simulink model "Scissor_Lift_2_Spring_Actuation"  (Simulink 7.9)
settings: Solver=ode15s  StartTime=0.0  StopTime=10.0  MaxStep=1e-2  RelTol=1e-3  AbsTol=1e-4
PostLoadFcn:
  | warning off mech2:compiler:topologyAnalysis:DanglingBlock
undefined symbols (not defined in the file): Local, Scissor_Lift_Param, X, Y, Z
libraries: sm_lib x46, Scissor_Parts_Lib x22, nesl_utility x3
(part 1 of 2)
Description:
  | Copyright 2012 The MathWorks, Inc.
settings Model: Creator=smiller  LastModifiedBy=smiller
settings ConfigurationSet: Description=SimMechanics 2G
settings ExplorerConfigSet: InternalSimMechanicsExplorerSettings="<ExplorerConfiguration><canonicalview>default</canonicalview><TilePanel><TileInfo><Tiles Columns=\"1\" Count=\"1\" Rows=\"1\"><Column Left=\"2\" Weight=\"1\"/><Column Left=\"398\"/><Row Top=\"2\" Weight=\"1\"/><Row Top=\"485\"/><Tile Height=\"1\" Width=\"1\" X=\"0\" Y=\"0\"/></Tiles></TileInfo><SceneInfo><SceneViewer><BGColor><R>0.60000002384185791</R><G>0.60000002384185791</G><B>0.60000002384185791</B></BGColor><Camera><Position><X>5.9281055778528522</X><Y>-5.497525414498786</Y><Z>4.0727654141199023</Z></Position><Center><X>1.3999999761581421</X><Y>0</Y><Z>1.5331412553787231</Z></Center><Up><X>-0.23055989473784222</X><Y>0.24511291789662082</Y><Z>0.94168030266045166</Z></Up><Left>-1.6471169292926788</Left><Right>1.6471169292926788</Right><Bottom>-2.5798462629318237</Bottom><Top>2.5798462629318237</Top></Camera></SceneViewer></SceneInfo></TilePanel></ExplorerConfiguration>"

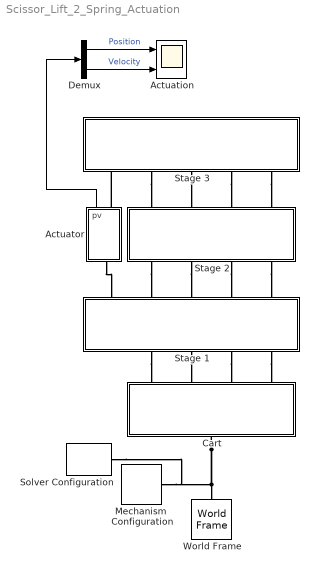
== system Scissor_Lift_2_Spring_Actuation ==
  Actuation : Scope  NumInputPorts=2
      settings: TimeRange=10  YMin=1.744052650646057~-0.2  YMax=2.541057843255645~0.3  SaveName=ScopeData3
  Actuator : Subsystem
  Cart : Subsystem
  Demux : Demux  Outputs=2
  Mechanism  Configuration : sm_lib/Utilities/Mechanism  Configuration  GravityVector=[0 0 -9.81]  GravityUnits=m/s^2  AllowGravitySignal=off  LinearizationDelta=0.001  BlockFunction=simmechanics.library.utilities.mechanism_configuration
  Solver Configuration : nesl_utility/Solver Configuration  PhysicalDomain=network_engine_domain  LeftPortType=input  RightPortType=generic  SubClassName=solver  UseCustomDae=off  DoDC=off  ResidualTolerance=1e-9  UseLocalSolver=off  LocalSolverChoice=NE_BACKWARD_EULER_ADVANCER  LocalSolverSampleTime=.001  DoFixedCost=off  MaxNonlinIter=3  MaxModeIter=2  LinearAlgebra=Sparse  Accelerate=off  Profile=off  UseLocalSampling=off  DelaysMemoryBudget=1024
  Stage 1 : Subsystem
  Stage 2 : Subsystem
  Stage 3 : Subsystem
  World Frame : sm_lib/Frames and  Transforms/World Frame  BlockFunction=simmechanics.library.frames_transforms.world_frame
  wires:
  Demux/1 -> Actuation/1  "Position"
  Demux/2 -> Actuation/2  "Velocity"
  Actuator/1(pv) -> Demux/1
  connections:
  Cart/LConn1 -- World Frame/RConn1 -- Solver Configuration/RConn1 -- Mechanism  Configuration/RConn1
  Stage 2/RConn1 -- Stage 1/LConn2
  Stage 2/RConn4 -- Stage 1/LConn5
  Stage 3/RConn2 -- Stage 2/LConn1
  Stage 2/RConn3 -- Stage 1/LConn4
  Stage 3/RConn4 -- Stage 2/LConn3
  Stage 3/RConn5 -- Stage 2/LConn4
  Stage 3/RConn3 -- Stage 2/LConn2
  Stage 1/RConn4 -- Cart/RConn3
  Stage 1/RConn3 -- Cart/RConn2
  Actuator/RConn1 -- Stage 3/RConn1
  Actuator/LConn1 -- Stage 1/LConn1
  Stage 1/RConn2 -- Cart/RConn1
  Stage 2/RConn2 -- Stage 1/LConn3
  Stage 1/RConn5 -- Cart/RConn4

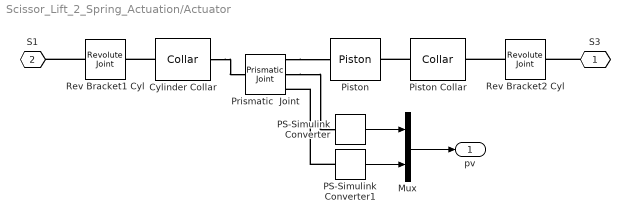
== system Scissor_Lift_2_Spring_Actuation/Actuator ==
  Cylinder Collar : Scissor_Parts_Lib/Collar  collar_length=Scissor_Lift_Param.Actuator.Collar.Length  collar_radius=Scissor_Lift_Param.Actuator.Collar.Radius  cylinder_length=Scissor_Lift_Param.Actuator.Cylinder.Length  cylinder_radius=Scissor_Lift_Param.Actuator.Cylinder.Radius  cylinder_ori=Local +Z  material_density=Scissor_Lift_Param.Actuator.Collar.Density  material_color=Scissor_Lift_Param.Actuator.Collar.Color  material_opacity=Scissor_Lift_Param.Actuator.Collar.Opacity
  Mux : Mux  Inputs=2
  PS-Simulink Converter : nesl_utility/PS-Simulink Converter  PhysicalDomain=network_engine_domain  LeftPortType=input  RightPortType=output  SubClassName=ps_output  Unit=1  AffineConversion=off
  PS-Simulink Converter1 : nesl_utility/PS-Simulink Converter  PhysicalDomain=network_engine_domain  LeftPortType=input  RightPortType=output  SubClassName=ps_output  Unit=1  AffineConversion=off
  Piston : Scissor_Parts_Lib/Piston  SystemSampleTime=-1
  Piston Collar : Scissor_Parts_Lib/Collar  collar_length=Scissor_Lift_Param.Actuator.Collar.Length  collar_radius=Scissor_Lift_Param.Actuator.Collar.Radius  cylinder_length=Scissor_Lift_Param.Actuator.Piston_Seat.Length  cylinder_radius=Scissor_Lift_Param.Actuator.Piston_Seat.Radius  cylinder_ori=Local -Z  material_density=Scissor_Lift_Param.Actuator.Collar.Density  material_color=Scissor_Lift_Param.Actuator.Collar.Color  material_opacity=Scissor_Lift_Param.Actuator.Collar.Opacity
  Prismatic  Joint : sm_lib/Joints/Prismatic  Joint  SenseConstraintForceX=off  SenseConstraintForceY=off  SenseConstraintForceZ=off  SenseConstraintTorqueX=off  SenseConstraintTorqueY=off  SenseConstraintTorqueZ=off  ConstraintWrenchDir=FollowerOnBase  ConstraintWrenchFrame=BaseFrame  EquilibriumPosition=Scissor_Lift_Param.Actuator.Spring.Equilibrium_Position  EquilibriumPositionUnits=cm  SpringStiffness=Scissor_Lift_Param.Actuator.Spring.Stiffness  SpringStiffnessUnits=N/m  DampingCoefficient=Scissor_Lift_Param.Actuator.Spring.Damping  DampingCoefficientUnits=N/(m/s)  ActuationMode=NoActuation  SensePosition=on  SenseVelocity=on  SenseAcceleration=off  SenseTorqueForce=off  PositionTargetValue=0  PositionTargetValueUnits=m  PositionTargetSpecify=off  PositionTargetPriority=High  VelocityTargetValue=0  VelocityTargetValueUnits=m/s  VelocityTargetSpecify=off  VelocityTargetPriority=High  BlockFunction=simmechanics.library.joints.prismatic_joint
  Rev Bracket1 Cyl : sm_lib/Joints/Revolute Joint  SenseConstraintForceX=off  SenseConstraintForceY=off  SenseConstraintForceZ=off  SenseConstraintTorqueX=off  SenseConstraintTorqueY=off  SenseConstraintTorqueZ=off  ConstraintWrenchDir=FollowerOnBase  ConstraintWrenchFrame=BaseFrame  EquilibriumPosition=0  EquilibriumPositionUnits=rad  SpringStiffness=0  SpringStiffnessUnits=N*m/rad  DampingCoefficient=0  DampingCoefficientUnits=N*m/(rad/s)  ActuationMode=NoActuation  SensePosition=off  SenseVelocity=off  SenseAcceleration=off  SenseTorqueForce=off  PositionTargetValue=0  PositionTargetValueUnits=rad  PositionTargetSpecify=off  PositionTargetPriority=High  VelocityTargetValue=0  VelocityTargetValueUnits=rad/s  VelocityTargetSpecify=off  VelocityTargetPriority=High  BlockFunction=simmechanics.library.joints.revolute_joint
  Rev Bracket2 Cyl : sm_lib/Joints/Revolute Joint  SenseConstraintForceX=off  SenseConstraintForceY=off  SenseConstraintForceZ=off  SenseConstraintTorqueX=off  SenseConstraintTorqueY=off  SenseConstraintTorqueZ=off  ConstraintWrenchDir=FollowerOnBase  ConstraintWrenchFrame=BaseFrame  EquilibriumPosition=0  EquilibriumPositionUnits=rad  SpringStiffness=0  SpringStiffnessUnits=N*m/rad  DampingCoefficient=0  DampingCoefficientUnits=N*m/(rad/s)  ActuationMode=NoActuation  SensePosition=off  SenseVelocity=off  SenseAcceleration=off  SenseTorqueForce=off  PositionTargetValue=0  PositionTargetValueUnits=rad  PositionTargetSpecify=off  PositionTargetPriority=High  VelocityTargetValue=0  VelocityTargetValueUnits=rad/s  VelocityTargetSpecify=off  VelocityTargetPriority=High  BlockFunction=simmechanics.library.joints.revolute_joint
  S3 : PMIOPort  Port=1  Side=Right
  S1 : PMIOPort  Port=2  Side=Left
  pv : Outport
  wires:
  Mux/1 -> pv/1
  PS-Simulink Converter1/1 -> Mux/2
  PS-Simulink Converter/1 -> Mux/1
  connections:
  PS-Simulink Converter1/LConn1 -- Prismatic  Joint/RConn3
  Prismatic  Joint/RConn2 -- PS-Simulink Converter/LConn1
  Rev Bracket1 Cyl/LConn1 -- S1/RConn1
  S3/RConn1 -- Rev Bracket2 Cyl/LConn1
  Rev Bracket2 Cyl/RConn1 -- Piston Collar/LConn1
  Piston Collar/RConn1 -- Piston/LConn1
  Prismatic  Joint/RConn1 -- Piston/RConn1
  Cylinder Collar/RConn1 -- Prismatic  Joint/LConn1
  Cylinder Collar/LConn1 -- Rev Bracket1 Cyl/RConn1

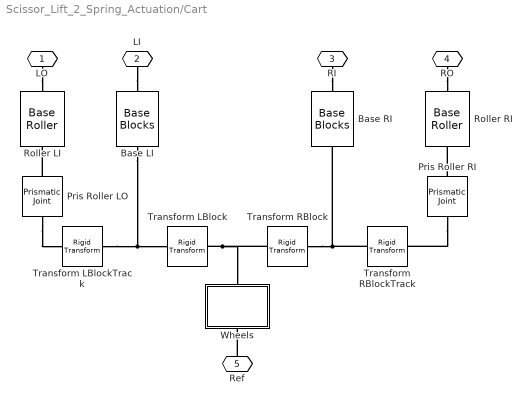
== system Scissor_Lift_2_Spring_Actuation/Cart ==
  Base LI : Scissor_Parts_Lib/Base Blocks  block_length=Scissor_Lift_Param.Base_Block.Length  block_width=Scissor_Lift_Param.Base_Block.Width  block_height=Scissor_Lift_Param.Base_Block.Height  shaft_radius=Scissor_Lift_Param.Roller.Shaft_Radius  shaft_length=Scissor_Lift_Param.Roller.Shaft_Length  material_density=Scissor_Lift_Param.Base_Block.Density  material_color=Scissor_Lift_Param.Base_Block.Color  material_opacity=Scissor_Lift_Param.Base_Block.Opacity
  Base RI : Scissor_Parts_Lib/Base Blocks  block_length=Scissor_Lift_Param.Base_Block.Length  block_width=Scissor_Lift_Param.Base_Block.Width  block_height=Scissor_Lift_Param.Base_Block.Height  shaft_radius=Scissor_Lift_Param.Roller.Shaft_Radius  shaft_length=Scissor_Lift_Param.Roller.Shaft_Length  material_density=Scissor_Lift_Param.Base_Block.Density  material_color=Scissor_Lift_Param.Base_Block.Color  material_opacity=Scissor_Lift_Param.Base_Block.Opacity
  Pris Roller LO : sm_lib/Joints/Prismatic  Joint  SenseConstraintForceX=off  SenseConstraintForceY=off  SenseConstraintForceZ=off  SenseConstraintTorqueX=off  SenseConstraintTorqueY=off  SenseConstraintTorqueZ=off  ConstraintWrenchDir=FollowerOnBase  ConstraintWrenchFrame=BaseFrame  EquilibriumPosition=0  EquilibriumPositionUnits=m  SpringStiffness=0  SpringStiffnessUnits=N/m  DampingCoefficient=0  DampingCoefficientUnits=N/(m/s)  ActuationMode=NoActuation  SensePosition=off  SenseVelocity=off  SenseAcceleration=off  SenseTorqueForce=off  PositionTargetValue=Scissor_Lift_Param.Roller.Init_Pos_Target  PositionTargetValueUnits=cm  PositionTargetSpecify=on  PositionTargetPriority=High  VelocityTargetValue=0  VelocityTargetValueUnits=m/s  VelocityTargetSpecify=off  VelocityTargetPriority=High  BlockFunction=simmechanics.library.joints.prismatic_joint
  Pris Roller RI : sm_lib/Joints/Prismatic  Joint  SenseConstraintForceX=off  SenseConstraintForceY=off  SenseConstraintForceZ=off  SenseConstraintTorqueX=off  SenseConstraintTorqueY=off  SenseConstraintTorqueZ=off  ConstraintWrenchDir=FollowerOnBase  ConstraintWrenchFrame=BaseFrame  EquilibriumPosition=0  EquilibriumPositionUnits=m  SpringStiffness=0  SpringStiffnessUnits=N/m  DampingCoefficient=0  DampingCoefficientUnits=N/(m/s)  ActuationMode=NoActuation  SensePosition=off  SenseVelocity=off  SenseAcceleration=off  SenseTorqueForce=off  PositionTargetValue=0  PositionTargetValueUnits=m  PositionTargetSpecify=off  PositionTargetPriority=High  VelocityTargetValue=0  VelocityTargetValueUnits=m/s  VelocityTargetSpecify=off  VelocityTargetPriority=High  BlockFunction=simmechanics.library.joints.prismatic_joint
  Roller LI : Scissor_Parts_Lib/Base Roller  roller_length=Scissor_Lift_Param.Roller.Roller_Length  roller_radius=Scissor_Lift_Param.Roller.Roller_Radius  shaft_length=Scissor_Lift_Param.Roller.Shaft_Length  shaft_radius=Scissor_Lift_Param.Roller.Shaft_Radius  material_density=Scissor_Lift_Param.Roller.Density  material_color=Scissor_Lift_Param.Roller.Color  material_opacity=Scissor_Lift_Param.Roller.Opacity
  Roller RI : Scissor_Parts_Lib/Base Roller  roller_length=Scissor_Lift_Param.Roller.Roller_Length  roller_radius=Scissor_Lift_Param.Roller.Roller_Radius  shaft_length=Scissor_Lift_Param.Roller.Shaft_Length  shaft_radius=Scissor_Lift_Param.Roller.Shaft_Radius  material_density=Scissor_Lift_Param.Roller.Density  material_color=Scissor_Lift_Param.Roller.Color  material_opacity=Scissor_Lift_Param.Roller.Opacity
  Transform LBlock : sm_lib/Frames and  Transforms/Rigid  Transform  TranslationMethod=Cartesian  TranslationLengthUnit=cm  TranslationStandardAxis=+Y  TranslationStandardOffset=Scissor_Lift_Param.Cart.Platform.Height/2  TranslationCartesianOffset=[20 0 Scissor_Lift_Param.Link_Separation.Outer_Outer/2-Scissor_Lift_Param.Link_Separation.Outer_Inner]  TranslationROffset=0  TranslationROffsetUnits=m  TranslationZOffset=0  TranslationZOffsetUnits=m  TranslationThetaOffset=0  TranslationThetaOffsetUnits=deg  RotationMethod=None  RotationAngleUnits=deg  RotationStandardAxis=+X  RotationAngle=90  RotationArbitraryAxis=[0 0 1]  FollAlignAxisA=+X  BaseAlignAxisA=+Y  FollAlignAxisB=+Y  BaseAlignAxisB=+Z  BlockFunction=simmechanics.library.frames_transforms.rigid_transform
  Transform LBlockTrack : sm_lib/Frames and  Transforms/Rigid  Transform  TranslationMethod=StandardAxis  TranslationLengthUnit=cm  TranslationStandardAxis=+Z  TranslationStandardOffset=Scissor_Lift_Param.Link_Separation.Outer_Inner  TranslationCartesianOffset=[0 0 0]  TranslationROffset=0  TranslationROffsetUnits=m  TranslationZOffset=0  TranslationZOffsetUnits=m  TranslationThetaOffset=0  TranslationThetaOffsetUnits=deg  RotationMethod=StandardAxis  RotationAngleUnits=deg  RotationStandardAxis=+Y  RotationAngle=90  RotationArbitraryAxis=[0 0 1]  FollAlignAxisA=+X  BaseAlignAxisA=+Y  FollAlignAxisB=+Y  BaseAlignAxisB=+Z  BlockFunction=simmechanics.library.frames_transforms.rigid_transform
  Transform RBlock : sm_lib/Frames and  Transforms/Rigid  Transform  TranslationMethod=Cartesian  TranslationLengthUnit=cm  TranslationStandardAxis=+Y  TranslationStandardOffset=Scissor_Lift_Param.Cart.Platform.Height/2  TranslationCartesianOffset=[20 0 -Scissor_Lift_Param.Link_Separation.Outer_Outer/2+Scissor_Lift_Param.Link_Separation.Outer_Inner]  TranslationROffset=0  TranslationROffsetUnits=m  TranslationZOffset=0  TranslationZOffsetUnits=m  TranslationThetaOffset=0  TranslationThetaOffsetUnits=deg  RotationMethod=None  RotationAngleUnits=deg  RotationStandardAxis=+X  RotationAngle=90  RotationArbitraryAxis=[0 0 1]  FollAlignAxisA=+X  BaseAlignAxisA=+Y  FollAlignAxisB=+Y  BaseAlignAxisB=+Z  BlockFunction=simmechanics.library.frames_transforms.rigid_transform
  Transform RBlockTrack : sm_lib/Frames and  Transforms/Rigid  Transform  TranslationMethod=StandardAxis  TranslationLengthUnit=cm  TranslationStandardAxis=-Z  TranslationStandardOffset=Scissor_Lift_Param.Link_Separation.Outer_Inner  TranslationCartesianOffset=[0 0 0]  TranslationROffset=0  TranslationROffsetUnits=m  TranslationZOffset=0  TranslationZOffsetUnits=m  TranslationThetaOffset=0  TranslationThetaOffsetUnits=deg  RotationMethod=StandardAxis  RotationAngleUnits=deg  RotationStandardAxis=+Y  RotationAngle=90  RotationArbitraryAxis=[0 0 1]  FollAlignAxisA=+X  BaseAlignAxisA=+Y  FollAlignAxisB=+Y  BaseAlignAxisB=+Z  BlockFunction=simmechanics.library.frames_transforms.rigid_transform
  Wheels : Subsystem
  LO : PMIOPort  Port=1  Side=Right
  LI : PMIOPort  Port=2  Side=Right
  RI : PMIOPort  Port=3  Side=Right
  RO : PMIOPort  Port=4  Side=Right
  Ref : PMIOPort  Port=5  Side=Left
  connections:
  Pris Roller LO/LConn1 -- Transform LBlockTrack/RConn1
  Pris Roller LO/RConn1 -- Roller LI/LConn1
  Transform LBlockTrack/LConn1 -- Base LI/LConn1 -- Transform LBlock/RConn1
  Transform RBlockTrack/LConn1 -- Base RI/LConn1 -- Transform RBlock/RConn1
  Pris Roller RI/LConn1 -- Transform RBlockTrack/RConn1
  Pris Roller RI/RConn1 -- Roller RI/LConn1
  Ref/RConn1 -- Wheels/LConn1
  LO/RConn1 -- Roller LI/RConn1
  LI/RConn1 -- Base LI/RConn1
  RO/RConn1 -- Roller RI/RConn1
  RI/RConn1 -- Base RI/RConn1
  Transform LBlock/LConn1 -- Wheels/RConn1 -- Transform RBlock/LConn1

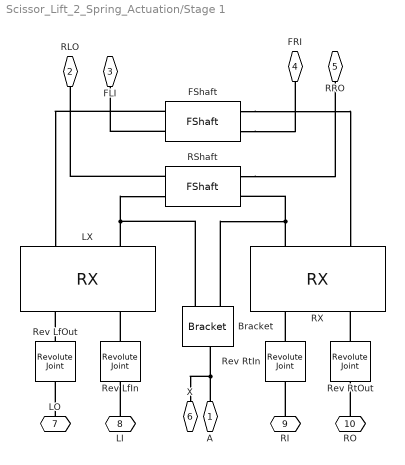
== system Scissor_Lift_2_Spring_Actuation/Stage 1 ==
  Bracket : Scissor_Parts_Lib/Bracket  fl_w=Scissor_Lift_Param.Actuator.Bracket.Flange.Width  fl_h=Scissor_Lift_Param.Actuator.Bracket.Flange.Height  T=Scissor_Lift_Param.Actuator.Bracket.Flange.Thickness  W=Scissor_Lift_Param.Actuator.Bracket.Flange.Offset  flupdown=Down  flfrontrear=Rear  fl_density=Scissor_Lift_Param.Actuator.Bracket.Flange.Density  fl_clr=Scissor_Lift_Param.Actuator.Bracket.Flange.Color  fl_opc=Scissor_Lift_Param.Actuator.Bracket.Flange.Opacity  shaft_length=Scissor_Lift_Param.Link_Separation.Outer_Outer-Scissor_Lift_Param.Link_Separation.Outer_Inner*2  shaft_radius=Scissor_Lift_Param.Actuator.Bracket.Shaft.Radius  shaft_density=Scissor_Lift_Param.Actuator.Bracket.Shaft.Density  shaft_color=Scissor_Lift_Param.Actuator.Bracket.Shaft.Color  shaft_opacity=Scissor_Lift_Param.Actuator.Bracket.Shaft.Opacity
  FShaft : Scissor_Parts_Lib/FShaft  sep_outer_outer=Scissor_Lift_Param.Link_Separation.Outer_Outer  sep_outer_inner=Scissor_Lift_Param.Link_Separation.Outer_Inner  shaft_radius=Scissor_Lift_Param.Trans_Shaft.Radius  shaft_density=Scissor_Lift_Param.Trans_Shaft.Density  shaft_color=Scissor_Lift_Param.Trans_Shaft.Color  shaft_opacity=Scissor_Lift_Param.Trans_Shaft.Opacity
  LX : Scissor_Parts_Lib/RX  link_length=Scissor_Lift_Param.Link.Length  link_width=Scissor_Lift_Param.Link.Width  link_thickness=Scissor_Lift_Param.Link.Thickness  link_hole_radius=Scissor_Lift_Param.Link.Hole_Radius  link_density=Scissor_Lift_Param.Link.Density  link_color=Scissor_Lift_Param.Link.Color  link_opacity=Scissor_Lift_Param.Link.Opacity  shaft_length=Scissor_Lift_Param.Link_Separation.Outer_Inner  shaft_radius=Scissor_Lift_Param.Link_Pin.Radius  shaft_density=Scissor_Lift_Param.Link_Pin.Density  shaft_color=Scissor_Lift_Param.Link_Pin.Color  shaft_opacity=Scissor_Lift_Param.Link_Pin.Opacity  leftright=Left  imgfile=Crossbar_RX_IMAGE.jpg  L1Port=OU  L2Port=IU  R1Port=OL  R2Port=IL
  RShaft : Scissor_Parts_Lib/FShaft  sep_outer_outer=Scissor_Lift_Param.Link_Separation.Outer_Outer  sep_outer_inner=Scissor_Lift_Param.Link_Separation.Outer_Inner  shaft_radius=Scissor_Lift_Param.Trans_Shaft.Radius  shaft_density=Scissor_Lift_Param.Trans_Shaft.Density  shaft_color=Scissor_Lift_Param.Trans_Shaft.Color  shaft_opacity=Scissor_Lift_Param.Trans_Shaft.Opacity
  RX : Scissor_Parts_Lib/RX  link_length=Scissor_Lift_Param.Link.Length  link_width=Scissor_Lift_Param.Link.Width  link_thickness=Scissor_Lift_Param.Link.Thickness  link_hole_radius=Scissor_Lift_Param.Link.Hole_Radius  link_density=Scissor_Lift_Param.Link.Density  link_color=Scissor_Lift_Param.Link.Color  link_opacity=Scissor_Lift_Param.Link.Opacity  shaft_length=Scissor_Lift_Param.Link_Separation.Outer_Inner  shaft_radius=Scissor_Lift_Param.Link_Pin.Radius  shaft_density=Scissor_Lift_Param.Link_Pin.Density  shaft_color=Scissor_Lift_Param.Link_Pin.Color  shaft_opacity=Scissor_Lift_Param.Link_Pin.Opacity  leftright=Right  imgfile=Crossbar_RX_IMAGE.jpg  L1Port=OU  L2Port=IU  R1Port=OL  R2Port=IL
  Rev LfIn : sm_lib/Joints/Revolute Joint  SenseConstraintForceX=off  SenseConstraintForceY=off  SenseConstraintForceZ=off  SenseConstraintTorqueX=off  SenseConstraintTorqueY=off  SenseConstraintTorqueZ=off  ConstraintWrenchDir=FollowerOnBase  ConstraintWrenchFrame=BaseFrame  EquilibriumPosition=0  EquilibriumPositionUnits=rad  SpringStiffness=0  SpringStiffnessUnits=N*m/rad  DampingCoefficient=0  DampingCoefficientUnits=N*m/(rad/s)  ActuationMode=NoActuation  SensePosition=off  SenseVelocity=off  SenseAcceleration=off  SenseTorqueForce=off  PositionTargetValue=0  PositionTargetValueUnits=deg  PositionTargetSpecify=off  PositionTargetPriority=Low  VelocityTargetValue=0  VelocityTargetValueUnits=rad/s  VelocityTargetSpecify=off  VelocityTargetPriority=High  BlockFunction=simmechanics.library.joints.revolute_joint
  Rev LfOut : sm_lib/Joints/Revolute Joint  SenseConstraintForceX=off  SenseConstraintForceY=off  SenseConstraintForceZ=off  SenseConstraintTorqueX=off  SenseConstraintTorqueY=off  SenseConstraintTorqueZ=off  ConstraintWrenchDir=FollowerOnBase  ConstraintWrenchFrame=BaseFrame  EquilibriumPosition=0  EquilibriumPositionUnits=rad  SpringStiffness=0  SpringStiffnessUnits=N*m/rad  DampingCoefficient=0  DampingCoefficientUnits=N*m/(rad/s)  ActuationMode=NoActuation  SensePosition=off  SenseVelocity=off  SenseAcceleration=off  SenseTorqueForce=off  PositionTargetValue=Scissor_Lift_Param.Crossbar.Init_Angle_Target  PositionTargetValueUnits=deg  PositionTargetSpecify=on  PositionTargetPriority=Low  VelocityTargetValue=0  VelocityTargetValueUnits=rad/s  VelocityTargetSpecify=off  VelocityTargetPriority=High  BlockFunction=simmechanics.library.joints.revolute_joint
  Rev RtIn : sm_lib/Joints/Revolute Joint  SenseConstraintForceX=off  SenseConstraintForceY=off  SenseConstraintForceZ=off  SenseConstraintTorqueX=off  SenseConstraintTorqueY=off  SenseConstraintTorqueZ=off  ConstraintWrenchDir=FollowerOnBase  ConstraintWrenchFrame=BaseFrame  EquilibriumPosition=0  EquilibriumPositionUnits=rad  SpringStiffness=0  SpringStiffnessUnits=N*m/rad  DampingCoefficient=0  DampingCoefficientUnits=N*m/(rad/s)  ActuationMode=NoActuation  SensePosition=off  SenseVelocity=off  SenseAcceleration=off  SenseTorqueForce=off  PositionTargetValue=0  PositionTargetValueUnits=deg  PositionTargetSpecify=off  PositionTargetPriority=Low  VelocityTargetValue=0  VelocityTargetValueUnits=rad/s  VelocityTargetSpecify=off  VelocityTargetPriority=High  BlockFunction=simmechanics.library.joints.revolute_joint
  Rev RtOut : sm_lib/Joints/Revolute Joint  SenseConstraintForceX=off  SenseConstraintForceY=off  SenseConstraintForceZ=off  SenseConstraintTorqueX=off  SenseConstraintTorqueY=off  SenseConstraintTorqueZ=off  ConstraintWrenchDir=FollowerOnBase  ConstraintWrenchFrame=BaseFrame  EquilibriumPosition=0  EquilibriumPositionUnits=rad  SpringStiffness=0  SpringStiffnessUnits=N*m/rad  DampingCoefficient=0  DampingCoefficientUnits=N*m/(rad/s)  ActuationMode=NoActuation  SensePosition=off  SenseVelocity=off  SenseAcceleration=off  SenseTorqueForce=off  PositionTargetValue=0  PositionTargetValueUnits=deg  PositionTargetSpecify=off  PositionTargetPriority=Low  VelocityTargetValue=0  VelocityTargetValueUnits=rad/s  VelocityTargetSpecify=off  VelocityTargetPriority=High  BlockFunction=simmechanics.library.joints.revolute_joint
  A : PMIOPort  Port=1  Side=Left
  RLO : PMIOPort  Port=2  Side=Left
  FLI : PMIOPort  Port=3  Side=Left
  FRI : PMIOPort  Port=4  Side=Left
  RRO : PMIOPort  Port=5  Side=Left
  X : PMIOPort  Port=6  Side=Right
  LO : PMIOPort  Port=7  Side=Right
  LI : PMIOPort  Port=8  Side=Right
  RI : PMIOPort  Port=9  Side=Right
  RO : PMIOPort  Port=10  Side=Right
  connections:
  A/RConn1 -- X/RConn1 -- Bracket/LConn1
  RO/RConn1 -- Rev RtOut/LConn1
  RI/RConn1 -- Rev RtIn/LConn1
  LO/RConn1 -- Rev LfOut/LConn1
  LI/RConn1 -- Rev LfIn/LConn1
  Rev RtOut/RConn1 -- RX/RConn2
  Rev RtIn/RConn1 -- RX/RConn1
  Bracket/RConn2 -- RShaft/RConn2 -- RX/LConn1
  RShaft/RConn1 -- RRO/RConn1
  RShaft/LConn1 -- RLO/RConn1
  Rev LfIn/RConn1 -- LX/RConn2
  Rev LfOut/RConn1 -- LX/RConn1
  Bracket/RConn1 -- RShaft/LConn2 -- LX/LConn2
  FShaft/RConn2 -- FRI/RConn1
  FShaft/RConn1 -- RX/LConn2
  FShaft/LConn2 -- FLI/RConn1
  FShaft/LConn1 -- LX/LConn1

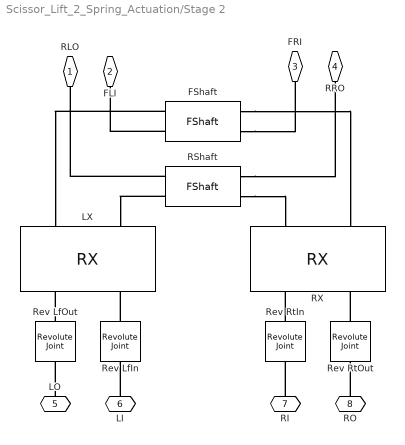
== system Scissor_Lift_2_Spring_Actuation/Stage 2 ==
  FShaft : Scissor_Parts_Lib/FShaft  sep_outer_outer=Scissor_Lift_Param.Link_Separation.Outer_Outer  sep_outer_inner=Scissor_Lift_Param.Link_Separation.Outer_Inner  shaft_radius=Scissor_Lift_Param.Trans_Shaft.Radius  shaft_density=Scissor_Lift_Param.Trans_Shaft.Density  shaft_color=Scissor_Lift_Param.Trans_Shaft.Color  shaft_opacity=Scissor_Lift_Param.Trans_Shaft.Opacity
  LX : Scissor_Parts_Lib/RX  link_length=Scissor_Lift_Param.Link.Length  link_width=Scissor_Lift_Param.Link.Width  link_thickness=Scissor_Lift_Param.Link.Thickness  link_hole_radius=Scissor_Lift_Param.Link.Hole_Radius  link_density=Scissor_Lift_Param.Link.Density  link_color=Scissor_Lift_Param.Link.Color  link_opacity=Scissor_Lift_Param.Link.Opacity  shaft_length=Scissor_Lift_Param.Link_Separation.Outer_Inner  shaft_radius=Scissor_Lift_Param.Link_Pin.Radius  shaft_density=Scissor_Lift_Param.Link_Pin.Density  shaft_color=Scissor_Lift_Param.Link_Pin.Color  shaft_opacity=Scissor_Lift_Param.Link_Pin.Opacity  leftright=Left  imgfile=Crossbar_RX_IMAGE.jpg  L1Port=OU  L2Port=IU  R1Port=OL  R2Port=IL
  RShaft : Scissor_Parts_Lib/FShaft  sep_outer_outer=Scissor_Lift_Param.Link_Separation.Outer_Outer  sep_outer_inner=Scissor_Lift_Param.Link_Separation.Outer_Inner  shaft_radius=Scissor_Lift_Param.Trans_Shaft.Radius  shaft_density=Scissor_Lift_Param.Trans_Shaft.Density  shaft_color=Scissor_Lift_Param.Trans_Shaft.Color  shaft_opacity=Scissor_Lift_Param.Trans_Shaft.Opacity
  RX : Scissor_Parts_Lib/RX  link_length=Scissor_Lift_Param.Link.Length  link_width=Scissor_Lift_Param.Link.Width  link_thickness=Scissor_Lift_Param.Link.Thickness  link_hole_radius=Scissor_Lift_Param.Link.Hole_Radius  link_density=Scissor_Lift_Param.Link.Density  link_color=Scissor_Lift_Param.Link.Color  link_opacity=Scissor_Lift_Param.Link.Opacity  shaft_length=Scissor_Lift_Param.Link_Separation.Outer_Inner  shaft_radius=Scissor_Lift_Param.Link_Pin.Radius  shaft_density=Scissor_Lift_Param.Link_Pin.Density  shaft_color=Scissor_Lift_Param.Link_Pin.Color  shaft_opacity=Scissor_Lift_Param.Link_Pin.Opacity  leftright=Right  imgfile=Crossbar_RX_IMAGE.jpg  L1Port=OU  L2Port=IU  R1Port=OL  R2Port=IL
  Rev LfIn : sm_lib/Joints/Revolute Joint  SenseConstraintForceX=off  SenseConstraintForceY=off  SenseConstraintForceZ=off  SenseConstraintTorqueX=off  SenseConstraintTorqueY=off  SenseConstraintTorqueZ=off  ConstraintWrenchDir=FollowerOnBase  ConstraintWrenchFrame=BaseFrame  EquilibriumPosition=0  EquilibriumPositionUnits=rad  SpringStiffness=0  SpringStiffnessUnits=N*m/rad  DampingCoefficient=0  DampingCoefficientUnits=N*m/(rad/s)  ActuationMode=NoActuation  SensePosition=off  SenseVelocity=off  SenseAcceleration=off  SenseTorqueForce=off  PositionTargetValue=0  PositionTargetValueUnits=deg  PositionTargetSpecify=off  PositionTargetPriority=Low  VelocityTargetValue=0  VelocityTargetValueUnits=rad/s  VelocityTargetSpecify=off  VelocityTargetPriority=High  BlockFunction=simmechanics.library.joints.revolute_joint
  Rev LfOut : sm_lib/Joints/Revolute Joint  SenseConstraintForceX=off  SenseConstraintForceY=off  SenseConstraintForceZ=off  SenseConstraintTorqueX=off  SenseConstraintTorqueY=off  SenseConstraintTorqueZ=off  ConstraintWrenchDir=FollowerOnBase  ConstraintWrenchFrame=BaseFrame  EquilibriumPosition=0  EquilibriumPositionUnits=rad  SpringStiffness=0  SpringStiffnessUnits=N*m/rad  DampingCoefficient=0  DampingCoefficientUnits=N*m/(rad/s)  ActuationMode=NoActuation  SensePosition=off  SenseVelocity=off  SenseAcceleration=off  SenseTorqueForce=off  PositionTargetValue=2*Scissor_Lift_Param.Crossbar.Init_Angle_Target  PositionTargetValueUnits=deg  PositionTargetSpecify=on  PositionTargetPriority=Low  VelocityTargetValue=0  VelocityTargetValueUnits=rad/s  VelocityTargetSpecify=off  VelocityTargetPriority=High  BlockFunction=simmechanics.library.joints.revolute_joint
  Rev RtIn : sm_lib/Joints/Revolute Joint  SenseConstraintForceX=off  SenseConstraintForceY=off  SenseConstraintForceZ=off  SenseConstraintTorqueX=off  SenseConstraintTorqueY=off  SenseConstraintTorqueZ=off  ConstraintWrenchDir=FollowerOnBase  ConstraintWrenchFrame=BaseFrame  EquilibriumPosition=0  EquilibriumPositionUnits=rad  SpringStiffness=0  SpringStiffnessUnits=N*m/rad  DampingCoefficient=0  DampingCoefficientUnits=N*m/(rad/s)  ActuationMode=NoActuation  SensePosition=off  SenseVelocity=off  SenseAcceleration=off  SenseTorqueForce=off  PositionTargetValue=0  PositionTargetValueUnits=deg  PositionTargetSpecify=off  PositionTargetPriority=Low  VelocityTargetValue=0  VelocityTargetValueUnits=rad/s  VelocityTargetSpecify=off  VelocityTargetPriority=High  BlockFunction=simmechanics.library.joints.revolute_joint
  Rev RtOut : sm_lib/Joints/Revolute Joint  SenseConstraintForceX=off  SenseConstraintForceY=off  SenseConstraintForceZ=off  SenseConstraintTorqueX=off  SenseConstraintTorqueY=off  SenseConstraintTorqueZ=off  ConstraintWrenchDir=FollowerOnBase  ConstraintWrenchFrame=BaseFrame  EquilibriumPosition=0  EquilibriumPositionUnits=rad  SpringStiffness=0  SpringStiffnessUnits=N*m/rad  DampingCoefficient=0  DampingCoefficientUnits=N*m/(rad/s)  ActuationMode=NoActuation  SensePosition=off  SenseVelocity=off  SenseAcceleration=off  SenseTorqueForce=off  PositionTargetValue=0  PositionTargetValueUnits=deg  PositionTargetSpecify=off  PositionTargetPriority=Low  VelocityTargetValue=0  VelocityTargetValueUnits=rad/s  VelocityTargetSpecify=off  VelocityTargetPriority=High  BlockFunction=simmechanics.library.joints.revolute_joint
  RLO : PMIOPort  Port=1  Side=Left
  FLI : PMIOPort  Port=2  Side=Left
  FRI : PMIOPort  Port=3  Side=Left
  RRO : PMIOPort  Port=4  Side=Left
  LO : PMIOPort  Port=5  Side=Right
  LI : PMIOPort  Port=6  Side=Right
  RI : PMIOPort  Port=7  Side=Right
  RO : PMIOPort  Port=8  Side=Right
  connections:
  FShaft/LConn1 -- LX/LConn1
  FShaft/LConn2 -- FLI/RConn1
  FShaft/RConn1 -- RX/LConn2
  FShaft/RConn2 -- FRI/RConn1
  RShaft/LConn2 -- LX/LConn2
  Rev LfOut/RConn1 -- LX/RConn1
  Rev LfIn/RConn1 -- LX/RConn2
  RShaft/LConn1 -- RLO/RConn1
  RShaft/RConn1 -- RRO/RConn1
  RShaft/RConn2 -- RX/LConn1
  Rev RtIn/RConn1 -- RX/RConn1
  Rev RtOut/RConn1 -- RX/RConn2
  LI/RConn1 -- Rev LfIn/LConn1
  LO/RConn1 -- Rev LfOut/LConn1
  RI/RConn1 -- Rev RtIn/LConn1
  RO/RConn1 -- Rev RtOut/LConn1

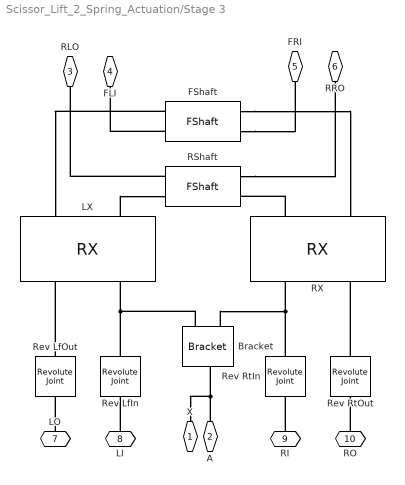
== system Scissor_Lift_2_Spring_Actuation/Stage 3 ==
  Bracket : Scissor_Parts_Lib/Bracket  fl_w=Scissor_Lift_Param.Actuator.Bracket.Flange.Width  fl_h=Scissor_Lift_Param.Actuator.Bracket.Flange.Height  T=Scissor_Lift_Param.Actuator.Bracket.Flange.Thickness  W=Scissor_Lift_Param.Actuator.Bracket.Flange.Offset  flupdown=Up  flfrontrear=Front  fl_density=Scissor_Lift_Param.Actuator.Bracket.Flange.Density  fl_clr=Scissor_Lift_Param.Actuator.Bracket.Flange.Color  fl_opc=Scissor_Lift_Param.Actuator.Bracket.Flange.Opacity  shaft_length=Scissor_Lift_Param.Link_Separation.Outer_Outer-Scissor_Lift_Param.Link_Separation.Outer_Inner*2  shaft_radius=Scissor_Lift_Param.Actuator.Bracket.Shaft.Radius  shaft_density=Scissor_Lift_Param.Actuator.Bracket.Shaft.Density  shaft_color=Scissor_Lift_Param.Actuator.Bracket.Shaft.Color  shaft_opacity=Scissor_Lift_Param.Actuator.Bracket.Shaft.Opacity
  FShaft : Scissor_Parts_Lib/FShaft  sep_outer_outer=Scissor_Lift_Param.Link_Separation.Outer_Outer  sep_outer_inner=Scissor_Lift_Param.Link_Separation.Outer_Inner  shaft_radius=Scissor_Lift_Param.Trans_Shaft.Radius  shaft_density=Scissor_Lift_Param.Trans_Shaft.Density  shaft_color=Scissor_Lift_Param.Trans_Shaft.Color  shaft_opacity=Scissor_Lift_Param.Trans_Shaft.Opacity
  LX : Scissor_Parts_Lib/RX  link_length=Scissor_Lift_Param.Link.Length  link_width=Scissor_Lift_Param.Link.Width  link_thickness=Scissor_Lift_Param.Link.Thickness  link_hole_radius=Scissor_Lift_Param.Link.Hole_Radius  link_density=Scissor_Lift_Param.Link.Density  link_color=Scissor_Lift_Param.Link.Color  link_opacity=Scissor_Lift_Param.Link.Opacity  shaft_length=Scissor_Lift_Param.Link_Separation.Outer_Inner  shaft_radius=Scissor_Lift_Param.Link_Pin.Radius  shaft_density=Scissor_Lift_Param.Link_Pin.Density  shaft_color=Scissor_Lift_Param.Link_Pin.Color  shaft_opacity=Scissor_Lift_Param.Link_Pin.Opacity  leftright=Left  imgfile=Crossbar_RX_IMAGE.jpg  L1Port=OU  L2Port=IU  R1Port=OL  R2Port=IL
  RShaft : Scissor_Parts_Lib/FShaft  sep_outer_outer=Scissor_Lift_Param.Link_Separation.Outer_Outer  sep_outer_inner=Scissor_Lift_Param.Link_Separation.Outer_Inner  shaft_radius=Scissor_Lift_Param.Trans_Shaft.Radius  shaft_density=Scissor_Lift_Param.Trans_Shaft.Density  shaft_color=Scissor_Lift_Param.Trans_Shaft.Color  shaft_opacity=Scissor_Lift_Param.Trans_Shaft.Opacity
  RX : Scissor_Parts_Lib/RX  link_length=Scissor_Lift_Param.Link.Length  link_width=Scissor_Lift_Param.Link.Width  link_thickness=Scissor_Lift_Param.Link.Thickness  link_hole_radius=Scissor_Lift_Param.Link.Hole_Radius  link_density=Scissor_Lift_Param.Link.Density  link_color=Scissor_Lift_Param.Link.Color  link_opacity=Scissor_Lift_Param.Link.Opacity  shaft_length=Scissor_Lift_Param.Link_Separation.Outer_Inner  shaft_radius=Scissor_Lift_Param.Link_Pin.Radius  shaft_density=Scissor_Lift_Param.Link_Pin.Density  shaft_color=Scissor_Lift_Param.Link_Pin.Color  shaft_opacity=Scissor_Lift_Param.Link_Pin.Opacity  leftright=Right  imgfile=Crossbar_RX_IMAGE.jpg  L1Port=OU  L2Port=IU  R1Port=OL  R2Port=IL
  Rev LfIn : sm_lib/Joints/Revolute Joint  SenseConstraintForceX=off  SenseConstraintForceY=off  SenseConstraintForceZ=off  SenseConstraintTorqueX=off  SenseConstraintTorqueY=off  SenseConstraintTorqueZ=off  ConstraintWrenchDir=FollowerOnBase  ConstraintWrenchFrame=BaseFrame  EquilibriumPosition=0  EquilibriumPositionUnits=rad  SpringStiffness=0  SpringStiffnessUnits=N*m/rad  DampingCoefficient=0  DampingCoefficientUnits=N*m/(rad/s)  ActuationMode=NoActuation  SensePosition=off  SenseVelocity=off  SenseAcceleration=off  SenseTorqueForce=off  PositionTargetValue=0  PositionTargetValueUnits=deg  PositionTargetSpecify=off  PositionTargetPriority=Low  VelocityTargetValue=0  VelocityTargetValueUnits=rad/s  VelocityTargetSpecify=off  VelocityTargetPriority=High  BlockFunction=simmechanics.library.joints.revolute_joint
  Rev LfOut : sm_lib/Joints/Revolute Joint  SenseConstraintForceX=off  SenseConstraintForceY=off  SenseConstraintForceZ=off  SenseConstraintTorqueX=off  SenseConstraintTorqueY=off  SenseConstraintTorqueZ=off  ConstraintWrenchDir=FollowerOnBase  ConstraintWrenchFrame=BaseFrame  EquilibriumPosition=0  EquilibriumPositionUnits=rad  SpringStiffness=0  SpringStiffnessUnits=N*m/rad  DampingCoefficient=0  DampingCoefficientUnits=N*m/(rad/s)  ActuationMode=NoActuation  SensePosition=off  SenseVelocity=off  SenseAcceleration=off  SenseTorqueForce=off  PositionTargetValue=2*Scissor_Lift_Param.Crossbar.Init_Angle_Target  PositionTargetValueUnits=deg  PositionTargetSpecify=on  PositionTargetPriority=Low  VelocityTargetValue=0  VelocityTargetValueUnits=rad/s  VelocityTargetSpecify=off  VelocityTargetPriority=High  BlockFunction=simmechanics.library.joints.revolute_joint
  Rev RtIn : sm_lib/Joints/Revolute Joint  SenseConstraintForceX=off  SenseConstraintForceY=off  SenseConstraintForceZ=off  SenseConstraintTorqueX=off  SenseConstraintTorqueY=off  SenseConstraintTorqueZ=off  ConstraintWrenchDir=FollowerOnBase  ConstraintWrenchFrame=BaseFrame  EquilibriumPosition=0  EquilibriumPositionUnits=rad  SpringStiffness=0  SpringStiffnessUnits=N*m/rad  DampingCoefficient=0  DampingCoefficientUnits=N*m/(rad/s)  ActuationMode=NoActuation  SensePosition=off  SenseVelocity=off  SenseAcceleration=off  SenseTorqueForce=off  PositionTargetValue=0  PositionTargetValueUnits=deg  PositionTargetSpecify=off  PositionTargetPriority=Low  VelocityTargetValue=0  VelocityTargetValueUnits=rad/s  VelocityTargetSpecify=off  VelocityTargetPriority=High  BlockFunction=simmechanics.library.joints.revolute_joint
  Rev RtOut : sm_lib/Joints/Revolute Joint  SenseConstraintForceX=off  SenseConstraintForceY=off  SenseConstraintForceZ=off  SenseConstraintTorqueX=off  SenseConstraintTorqueY=off  SenseConstraintTorqueZ=off  ConstraintWrenchDir=FollowerOnBase  ConstraintWrenchFrame=BaseFrame  EquilibriumPosition=0  EquilibriumPositionUnits=rad  SpringStiffness=0  SpringStiffnessUnits=N*m/rad  DampingCoefficient=0  DampingCoefficientUnits=N*m/(rad/s)  ActuationMode=NoActuation  SensePosition=off  SenseVelocity=off  SenseAcceleration=off  SenseTorqueForce=off  PositionTargetValue=0  PositionTargetValueUnits=deg  PositionTargetSpecify=off  PositionTargetPriority=Low  VelocityTargetValue=0  VelocityTargetValueUnits=rad/s  VelocityTargetSpecify=off  VelocityTargetPriority=High  BlockFunction=simmechanics.library.joints.revolute_joint
  X : PMIOPort  Port=1  Side=Left
  A : PMIOPort  Port=2  Side=Right
  RLO : PMIOPort  Port=3  Side=Left
  FLI : PMIOPort  Port=4  Side=Left
  FRI : PMIOPort  Port=5  Side=Left
  RRO : PMIOPort  Port=6  Side=Left
  LO : PMIOPort  Port=7  Side=Right
  LI : PMIOPort  Port=8  Side=Right
  RI : PMIOPort  Port=9  Side=Right
  RO : PMIOPort  Port=10  Side=Right
  connections:
  FShaft/LConn1 -- LX/LConn1
  FShaft/LConn2 -- FLI/RConn1
  FShaft/RConn1 -- RX/LConn2
  FShaft/RConn2 -- FRI/RConn1
  LX/LConn2 -- RShaft/LConn2
  Rev LfOut/RConn1 -- LX/RConn1
  Bracket/RConn1 -- LX/RConn2 -- Rev LfIn/RConn1
  RShaft/LConn1 -- RLO/RConn1
  RShaft/RConn1 -- RRO/RConn1
  RX/LConn1 -- RShaft/RConn2
  Bracket/RConn2 -- RX/RConn1 -- Rev RtIn/RConn1
  Rev RtOut/RConn1 -- RX/RConn2
  LI/RConn1 -- Rev LfIn/LConn1
  LO/RConn1 -- Rev LfOut/LConn1
  RI/RConn1 -- Rev RtIn/LConn1
  RO/RConn1 -- Rev RtOut/LConn1
  A/RConn1 -- Bracket/LConn1 -- X/RConn1

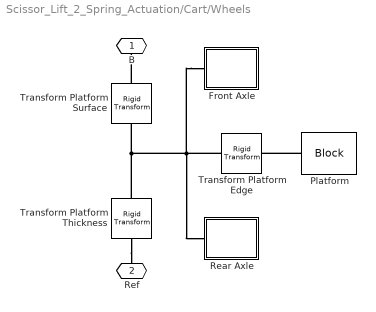
== system Scissor_Lift_2_Spring_Actuation/Cart/Wheels ==
  Front Axle : Subsystem
  Platform : Scissor_Parts_Lib/Block  L=Scissor_Lift_Param.Cart.Platform.Width  W=Scissor_Lift_Param.Cart.Platform.Length  H=Scissor_Lift_Param.Cart.Platform.Height  z_ori=Local +Z  rho=Scissor_Lift_Param.Base_Block.Density  clr=Scissor_Lift_Param.Base_Block.Color  opc=Scissor_Lift_Param.Base_Block.Opacity
  Rear Axle : Subsystem
  Transform Platform Surface : sm_lib/Frames and  Transforms/Rigid  Transform  TranslationMethod=Cartesian  TranslationLengthUnit=cm  TranslationStandardAxis=+Y  TranslationStandardOffset=Scissor_Lift_Param.Cart.Platform.Height/2  TranslationCartesianOffset=[0 Scissor_Lift_Param.Cart.Platform.Height/2 0]  TranslationROffset=0  TranslationROffsetUnits=m  TranslationZOffset=0  TranslationZOffsetUnits=m  TranslationThetaOffset=0  TranslationThetaOffsetUnits=deg  RotationMethod=None  RotationAngleUnits=deg  RotationStandardAxis=+X  RotationAngle=90  RotationArbitraryAxis=[0 0 1]  FollAlignAxisA=+X  BaseAlignAxisA=+Y  FollAlignAxisB=+Y  BaseAlignAxisB=+Z  BlockFunction=simmechanics.library.frames_transforms.rigid_transform
  Transform Platform Thickness : sm_lib/Frames and  Transforms/Rigid  Transform  TranslationMethod=StandardAxis  TranslationLengthUnit=cm  TranslationStandardAxis=+Z  TranslationStandardOffset=Scissor_Lift_Param.Cart.Platform.Height/2  TranslationCartesianOffset=[0 0 0]  TranslationROffset=0  TranslationROffsetUnits=m  TranslationZOffset=0  TranslationZOffsetUnits=m  TranslationThetaOffset=0  TranslationThetaOffsetUnits=deg  RotationMethod=StandardAxis  RotationAngleUnits=deg  RotationStandardAxis=+X  RotationAngle=90  RotationArbitraryAxis=[0 0 1]  FollAlignAxisA=+X  BaseAlignAxisA=+Y  FollAlignAxisB=+Y  BaseAlignAxisB=+Z  BlockFunction=simmechanics.library.frames_transforms.rigid_transform
  Transform Platform Edge : sm_lib/Frames and  Transforms/Rigid  Transform  TranslationMethod=Cartesian  TranslationLengthUnit=cm  TranslationStandardAxis=+Z  TranslationStandardOffset=0  TranslationCartesianOffset=[Scissor_Lift_Param.Cart.Platform.Length 0 -Scissor_Lift_Param.Cart.Platform.Width]/2  TranslationROffset=0  TranslationROffsetUnits=m  TranslationZOffset=0  TranslationZOffsetUnits=m  TranslationThetaOffset=0  TranslationThetaOffsetUnits=deg  RotationMethod=None  RotationAngleUnits=deg  RotationStandardAxis=+X  RotationAngle=90  RotationArbitraryAxis=[0 0 1]  FollAlignAxisA=+X  BaseAlignAxisA=+Y  FollAlignAxisB=+Y  BaseAlignAxisB=+Z  BlockFunction=simmechanics.library.frames_transforms.rigid_transform
  " B" : PMIOPort  Port=1  Side=Right
  Ref : PMIOPort  Port=2  Side=Left
  connections:
  Transform Platform Surface/RConn1 -- " B"/RConn1
  Transform Platform Thickness/LConn1 -- Ref/RConn1
  Platform/LConn1 -- Transform Platform Edge/RConn1
  Front Axle/LConn1 -- Rear Axle/LConn1 -- Transform Platform Surface/LConn1 -- Transform Platform Thickness/RConn1 -- Transform Platform Edge/LConn1

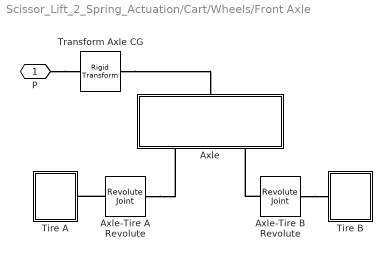
== system Scissor_Lift_2_Spring_Actuation/Cart/Wheels/Front Axle ==
  Axle : Subsystem  mask(Axle){Ra=Scissor_Lift_Param.Cart.Axle.Radius, Wd=Scissor_Lift_Param.Cart.Axle.Wheel_Distance, Rr=Scissor_Lift_Param.Cart.Axle.Rim.Radius, Tr=Scissor_Lift_Param.Cart.Axle.Rim.Thickness, rho=Scissor_Lift_Param.Cart.Axle.Rim.Density, clr=Scissor_Lift_Param.Cart.Axle.Rim.Color}
      mask prompts: Ra "Axle radius (cm)"; Wd "Wheel distance (cm)"; Rr "Rim radius (cm)"; Tr "Rim thickness (cm)"; rho "Density (kg/m^3)"; clr "Color"
      mask TabNameString: Dimensions,Dimensions,Dimensions,Dimensions,Material Properties,Material Properties
      mask Display:
      | image(imread('sm_wlandgear_axle.png'));
      | port_label('LConn',1,'M');
      | port_label('RConn',1,'L');
      | port_label('RConn',2,'R');
  Axle-Tire A Revolute : sm_lib/Joints/Revolute Joint  SenseConstraintForceX=off  SenseConstraintForceY=off  SenseConstraintForceZ=off  SenseConstraintTorqueX=off  SenseConstraintTorqueY=off  SenseConstraintTorqueZ=off  ConstraintWrenchDir=FollowerOnBase  ConstraintWrenchFrame=BaseFrame  EquilibriumPosition=0  EquilibriumPositionUnits=rad  SpringStiffness=0  SpringStiffnessUnits=N*m/rad  DampingCoefficient=0  DampingCoefficientUnits=N*m/(rad/s)  ActuationMode=NoActuation  SensePosition=off  SenseVelocity=off  SenseAcceleration=off  SenseTorqueForce=off  PositionTargetValue=0  PositionTargetValueUnits=rad  PositionTargetSpecify=off  PositionTargetPriority=High  VelocityTargetValue=0  VelocityTargetValueUnits=rad/s  VelocityTargetSpecify=off  VelocityTargetPriority=High  BlockFunction=simmechanics.library.joints.revolute_joint
  Axle-Tire B Revolute : sm_lib/Joints/Revolute Joint  SenseConstraintForceX=off  SenseConstraintForceY=off  SenseConstraintForceZ=off  SenseConstraintTorqueX=off  SenseConstraintTorqueY=off  SenseConstraintTorqueZ=off  ConstraintWrenchDir=FollowerOnBase  ConstraintWrenchFrame=BaseFrame  EquilibriumPosition=0  EquilibriumPositionUnits=rad  SpringStiffness=0  SpringStiffnessUnits=N*m/rad  DampingCoefficient=0  DampingCoefficientUnits=N*m/(rad/s)  ActuationMode=NoActuation  SensePosition=off  SenseVelocity=off  SenseAcceleration=off  SenseTorqueForce=off  PositionTargetValue=0  PositionTargetValueUnits=rad  PositionTargetSpecify=off  PositionTargetPriority=High  VelocityTargetValue=0  VelocityTargetValueUnits=rad/s  VelocityTargetSpecify=off  VelocityTargetPriority=High  BlockFunction=simmechanics.library.joints.revolute_joint
  Tire A : Subsystem  mask(Tire){Rt=Scissor_Lift_Param.Cart.Axle.Tire.Radius, Rr=Scissor_Lift_Param.Cart.Axle.Rim.Radius, Tt=Scissor_Lift_Param.Cart.Axle.Tire.Thickness, rho=Scissor_Lift_Param.Cart.Axle.Tire.Density, clr=Scissor_Lift_Param.Cart.Axle.Tire.Color}
      mask prompts: Rt "Tire radius (cm)"; Rr "Rim radius (cm)"; Tt "Tire thickness (cm)"; rho "Density (kg/m^3)"; clr "Color"
      mask init:
      | theta = [(0:1:359) 0]'*pi/180;
      | unit_circle = [cos(theta), sin(theta)];
      | tire_sec = [Rt * unit_circle; Rr * flipud(unit_circle)];
      mask TabNameString: Dimensions,Dimensions,Dimensions,Material Properties,Material Properties
      mask Display:
      | image(imread('sm_wlandgear_tire.png'));
      | port_label('LConn',1,'C');
  Tire B : Subsystem  mask(Tire){Rt=Scissor_Lift_Param.Cart.Axle.Tire.Radius, Rr=Scissor_Lift_Param.Cart.Axle.Rim.Radius, Tt=Scissor_Lift_Param.Cart.Axle.Tire.Thickness, rho=Scissor_Lift_Param.Cart.Axle.Tire.Density, clr=Scissor_Lift_Param.Cart.Axle.Tire.Color}
      mask prompts: Rt "Tire radius (cm)"; Rr "Rim radius (cm)"; Tt "Tire thickness (cm)"; rho "Density (kg/m^3)"; clr "Color"
      mask init:
      | theta = [(0:1:359) 0]'*pi/180;
      | unit_circle = [cos(theta), sin(theta)];
      | tire_sec = [Rt * unit_circle; Rr * flipud(unit_circle)];
      mask TabNameString: Dimensions,Dimensions,Dimensions,Material Properties,Material Properties
      mask Display:
      | image(imread('sm_wlandgear_tire.png'));
      | port_label('LConn',1,'C');
  Transform Axle CG : sm_lib/Frames and  Transforms/Rigid  Transform  TranslationMethod=Cartesian  TranslationLengthUnit=cm  TranslationStandardAxis=+Z  TranslationStandardOffset=0  TranslationCartesianOffset=[Scissor_Lift_Param.Cart.Axle.Tire.Radius+Scissor_Lift_Param.Cart.Axle.Wheelbase -Scissor_Lift_Param.Cart.Axle.Tire.Radius 0]  TranslationROffset=0  TranslationROffsetUnits=m  TranslationZOffset=0  TranslationZOffsetUnits=m  TranslationThetaOffset=0  TranslationThetaOffsetUnits=deg  RotationMethod=None  RotationAngleUnits=deg  RotationStandardAxis=+X  RotationAngle=90  RotationArbitraryAxis=[0 0 1]  FollAlignAxisA=+X  BaseAlignAxisA=+Y  FollAlignAxisB=+Y  BaseAlignAxisB=+Z  BlockFunction=simmechanics.library.frames_transforms.rigid_transform
  P : PMIOPort  Port=1  Side=Left
  connections:
  Axle-Tire A Revolute/LConn1 -- Axle/RConn1
  Axle-Tire A Revolute/RConn1 -- Tire A/LConn1
  Axle-Tire B Revolute/LConn1 -- Axle/RConn2
  Axle-Tire B Revolute/RConn1 -- Tire B/LConn1
  Transform Axle CG/RConn1 -- Axle/LConn1
  P/RConn1 -- Transform Axle CG/LConn1

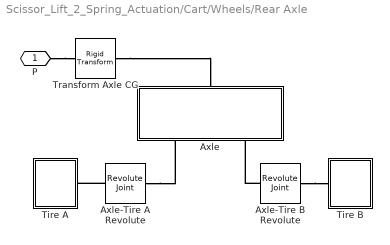
== system Scissor_Lift_2_Spring_Actuation/Cart/Wheels/Rear Axle ==
  Axle : Subsystem  mask(Axle){Ra=Scissor_Lift_Param.Cart.Axle.Radius, Wd=Scissor_Lift_Param.Cart.Axle.Wheel_Distance, Rr=Scissor_Lift_Param.Cart.Axle.Rim.Radius, Tr=Scissor_Lift_Param.Cart.Axle.Rim.Thickness, rho=Scissor_Lift_Param.Cart.Axle.Rim.Density, clr=Scissor_Lift_Param.Cart.Axle.Rim.Color}
      mask prompts: Ra "Axle radius (cm)"; Wd "Wheel distance (cm)"; Rr "Rim radius (cm)"; Tr "Rim thickness (cm)"; rho "Density (kg/m^3)"; clr "Color"
      mask TabNameString: Dimensions,Dimensions,Dimensions,Dimensions,Material Properties,Material Properties
      mask Display:
      | image(imread('sm_wlandgear_axle.png'));
      | port_label('LConn',1,'M');
      | port_label('RConn',1,'L');
      | port_label('RConn',2,'R');
  Axle-Tire A Revolute : sm_lib/Joints/Revolute Joint  SenseConstraintForceX=off  SenseConstraintForceY=off  SenseConstraintForceZ=off  SenseConstraintTorqueX=off  SenseConstraintTorqueY=off  SenseConstraintTorqueZ=off  ConstraintWrenchDir=FollowerOnBase  ConstraintWrenchFrame=BaseFrame  EquilibriumPosition=0  EquilibriumPositionUnits=rad  SpringStiffness=0  SpringStiffnessUnits=N*m/rad  DampingCoefficient=0  DampingCoefficientUnits=N*m/(rad/s)  ActuationMode=NoActuation  SensePosition=off  SenseVelocity=off  SenseAcceleration=off  SenseTorqueForce=off  PositionTargetValue=0  PositionTargetValueUnits=rad  PositionTargetSpecify=off  PositionTargetPriority=High  VelocityTargetValue=0  VelocityTargetValueUnits=rad/s  VelocityTargetSpecify=off  VelocityTargetPriority=High  BlockFunction=simmechanics.library.joints.revolute_joint
  Axle-Tire B Revolute : sm_lib/Joints/Revolute Joint  SenseConstraintForceX=off  SenseConstraintForceY=off  SenseConstraintForceZ=off  SenseConstraintTorqueX=off  SenseConstraintTorqueY=off  SenseConstraintTorqueZ=off  ConstraintWrenchDir=FollowerOnBase  ConstraintWrenchFrame=BaseFrame  EquilibriumPosition=0  EquilibriumPositionUnits=rad  SpringStiffness=0  SpringStiffnessUnits=N*m/rad  DampingCoefficient=0  DampingCoefficientUnits=N*m/(rad/s)  ActuationMode=NoActuation  SensePosition=off  SenseVelocity=off  SenseAcceleration=off  SenseTorqueForce=off  PositionTargetValue=0  PositionTargetValueUnits=rad  PositionTargetSpecify=off  PositionTargetPriority=High  VelocityTargetValue=0  VelocityTargetValueUnits=rad/s  VelocityTargetSpecify=off  VelocityTargetPriority=High  BlockFunction=simmechanics.library.joints.revolute_joint
  Tire A : Subsystem  mask(Tire){Rt=Scissor_Lift_Param.Cart.Axle.Tire.Radius, Rr=Scissor_Lift_Param.Cart.Axle.Rim.Radius, Tt=Scissor_Lift_Param.Cart.Axle.Tire.Thickness, rho=Scissor_Lift_Param.Cart.Axle.Tire.Density, clr=Scissor_Lift_Param.Cart.Axle.Tire.Color}
      mask prompts: Rt "Tire radius (cm)"; Rr "Rim radius (cm)"; Tt "Tire thickness (cm)"; rho "Density (kg/m^3)"; clr "Color"
      mask init:
      | theta = [(0:1:359) 0]'*pi/180;
      | unit_circle = [cos(theta), sin(theta)];
      | tire_sec = [Rt * unit_circle; Rr * flipud(unit_circle)];
      mask TabNameString: Dimensions,Dimensions,Dimensions,Material Properties,Material Properties
      mask Display:
      | image(imread('sm_wlandgear_tire.png'));
      | port_label('LConn',1,'C');
  Tire B : Subsystem  mask(Tire){Rt=Scissor_Lift_Param.Cart.Axle.Tire.Radius, Rr=Scissor_Lift_Param.Cart.Axle.Rim.Radius, Tt=Scissor_Lift_Param.Cart.Axle.Tire.Thickness, rho=Scissor_Lift_Param.Cart.Axle.Tire.Density, clr=Scissor_Lift_Param.Cart.Axle.Tire.Color}
      mask prompts: Rt "Tire radius (cm)"; Rr "Rim radius (cm)"; Tt "Tire thickness (cm)"; rho "Density (kg/m^3)"; clr "Color"
      mask init:
      | theta = [(0:1:359) 0]'*pi/180;
      | unit_circle = [cos(theta), sin(theta)];
      | tire_sec = [Rt * unit_circle; Rr * flipud(unit_circle)];
      mask TabNameString: Dimensions,Dimensions,Dimensions,Material Properties,Material Properties
      mask Display:
      | image(imread('sm_wlandgear_tire.png'));
      | port_label('LConn',1,'C');
  Transform Axle CG : sm_lib/Frames and  Transforms/Rigid  Transform  TranslationMethod=Cartesian  TranslationLengthUnit=cm  TranslationStandardAxis=+Z  TranslationStandardOffset=0  TranslationCartesianOffset=[Scissor_Lift_Param.Cart.Axle.Tire.Radius -Scissor_Lift_Param.Cart.Axle.Tire.Radius 0]  TranslationROffset=0  TranslationROffsetUnits=m  TranslationZOffset=0  TranslationZOffsetUnits=m  TranslationThetaOffset=0  TranslationThetaOffsetUnits=deg  RotationMethod=None  RotationAngleUnits=deg  RotationStandardAxis=+X  RotationAngle=90  RotationArbitraryAxis=[0 0 1]  FollAlignAxisA=+X  BaseAlignAxisA=+Y  FollAlignAxisB=+Y  BaseAlignAxisB=+Z  BlockFunction=simmechanics.library.frames_transforms.rigid_transform
  P : PMIOPort  Port=1  Side=Left
  connections:
  P/RConn1 -- Transform Axle CG/LConn1
  Transform Axle CG/RConn1 -- Axle/LConn1
  Axle-Tire A Revolute/RConn1 -- Tire A/LConn1
  Axle-Tire B Revolute/RConn1 -- Tire B/LConn1
  Axle-Tire B Revolute/LConn1 -- Axle/RConn2
  Axle-Tire A Revolute/LConn1 -- Axle/RConn1
